simulink model "sweep_mod1"  (Simulink 7.9)
settings: Solver=VariableStepDiscrete  StartTime=0.0  StopTime=simu.trantime  RelTol=1e-3
undefined symbols (not defined in the file): Fs, mod
libraries: dspsigops x2, dspsrcs4 x1
settings Model: Creator=Isacco Arnaldi  LastModifiedBy=Arnaldi Isacco
settings SolverCC: AutoInsertRateTranBlk=on
settings DataIOCC: LimitDataPoints=off  MaxDataPoints=50000  SaveOutput=off  SaveTime=off
settings OptimizationCC: InlineParams=on
settings DebuggingCC: SolverPrmCheckMsg=none  StrictBusMsg=Warning
settings CodeAppCC: CustomSymbolStrType=$N$R$M_T
settings GRTTargetCC: CombineOutputUpdateFcns=off  GRTInterface=on

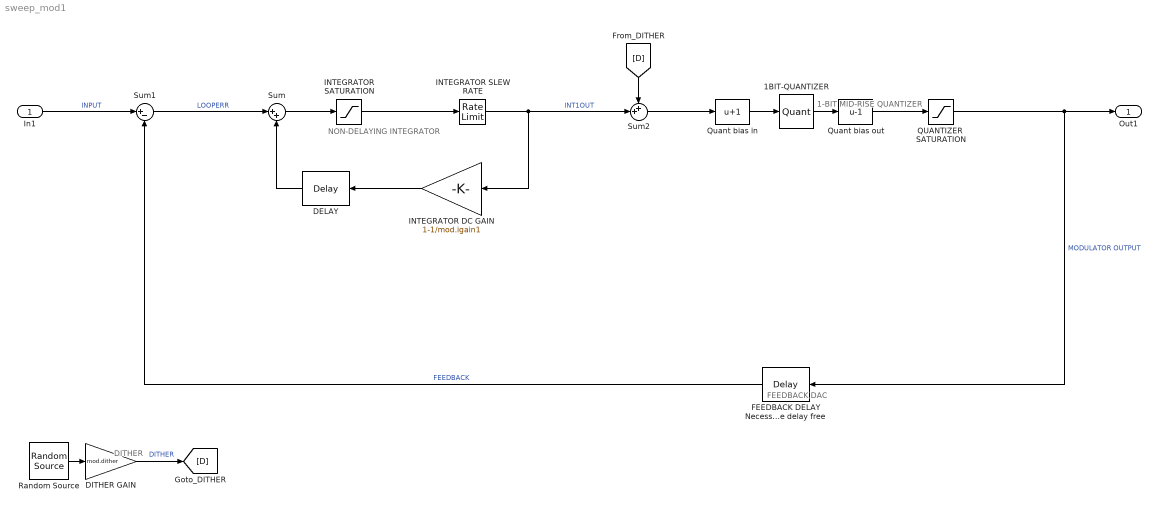
== system sweep_mod1 ==
  note: NON-DELAYING INTEGRATOR
  note: FEEDBACK DAC
  note: 1-BIT MID-RISE QUANTIZER
  note: DITHER
  In1 : Inport
  1BIT-QUANTIZER : Quantizer  QuantizationInterval=2  SampleTime=1/Fs
      settings: AttributesFormatString=step = 2
  DELAY : dspsigops/Delay  InputProcessing=Inherited (this choice will be removed - see release notes)  dly_unit=Samples  delay=1  ic_detail=off  dif_ic_for_ch=off  dif_ic_for_dly=off  ic=0  reset_popup=None
  DITHER GAIN : Gain  Gain=mod.dither  SampleTime=1/Fs
  FEEDBACK DELAY Necessary to avoid a delay-free loop as integrator and quantizer are delay free : dspsigops/Delay  InputProcessing=Inherited (this choice will be removed - see release notes)  dly_unit=Samples  delay=1  ic_detail=off  dif_ic_for_ch=off  dif_ic_for_dly=off  ic=0  reset_popup=None
  INTEGRATOR SATURATION : Saturate  UpperLimit=mod.isat1  LowerLimit=-(mod.isat1)  SampleTime=1/Fs
      settings: AttributesFormatString=Real integrators will have output\nswing limits (analog signal headroom\nor digital accumulator min/max values)
  INTEGRATOR SLEW RATE : RateLimiter  RisingSlewLimit=mod.isr1  FallingSlewLimit=-(mod.isr1)  SampleTimeMode=inherited
      settings: AttributesFormatString=...and may suffer from\npoor slew rate
  INTEGRATOR DC GAIN : Gain  Gain=1-1/mod.igain1  SampleTime=1/Fs
      settings: AttributesFormatString=Integrator leakage\n(model finite integrator dc/LF\ngain in analog modulators)
  QUANTIZER  SATURATION : Saturate  UpperLimit=mod.qsatout1  LowerLimit=-(mod.qsatout1)  SampleTime=1/Fs
      settings: AttributesFormatString=Limit quantizer\noutput
  Quant bias in : Bias  Bias=1
      settings: AttributesFormatString=Need offset to give\nMID-RISE quantiser
  Quant bias out : Bias  Bias=-1
      settings: AttributesFormatString=Shift outputs to\n..., -2, 1, 1, ...
  Random Source : dspsrcs4/Random Source  SrcType=Uniform  NormMethod=Ziggurat  CltLength=12  MinVal=-1  MaxVal=1  MeanVal=0  VarVal=1  RepMode=Not repeatable  rawSeed=1  IsInherit=off  SampMode=Discrete  SampTime=1/Fs  SampFrame=1  DataType=Double  OutComplex=Real
  Sum : Sum  Inputs=|++  SampleTime=1/Fs
      settings: AttributesFormatString=Integrator\nsummer
  Sum1 : Sum  Inputs=|+-  SampleTime=1/Fs
      settings: AttributesFormatString=Modulator Input\nLoop Error (input - fbk)
  Sum2 : Sum  Inputs=++|  SampleTime=1/Fs
  Out1 : Outport
  wires:
  DELAY/1 -> Sum/2
  Sum/1 -> INTEGRATOR SATURATION/1
  Sum1/1 -> Sum/1  "LOOPERR"
  FEEDBACK DELAY Necessary to avoid a delay-free loop as integrator and quantizer are delay free/1 -> Sum1/2  "FEEDBACK"
  Random Source/1 -> DITHER GAIN/1
  INTEGRATOR DC GAIN/1 -> DELAY/1
  Quant bias out/1 -> QUANTIZER  SATURATION/1
  DITHER GAIN/1 -> [D]  "DITHER"
  Quant bias in/1 -> 1BIT-QUANTIZER/1
  1BIT-QUANTIZER/1 -> Quant bias out/1
  Sum2/1 -> Quant bias in/1
  [D] -> Sum2/1
  INTEGRATOR SLEW RATE/1 -> INTEGRATOR DC GAIN/1, Sum2/2  "INT1OUT"
  INTEGRATOR SATURATION/1 -> INTEGRATOR SLEW RATE/1
  QUANTIZER  SATURATION/1 -> FEEDBACK DELAY Necessary to avoid a delay-free loop as integrator and quantizer are delay free/1, Out1/1  "MODULATOR OUTPUT"
  In1/1 -> Sum1/1  "INPUT"
